simulink model "SG__MDL_IO344"  (R2020a)
settings: Solver=FixedStepDiscrete  StartTime=0.0  StopTime=Inf  RelTol=1e-3  EnableMultiTasking=on
PreLoadFcn:
  | Ts = 0.001;
  | FPGA_Frequency = 75000000;
InitFcn:
  | Ts = 0.001;
  | FPGA_Frequency = 75000000;
libraries: dspfdesign x4, slrtlib x2, SG_library x1, simulink x1, dspsrcs4 x1
settings Model: SimulationMode=external  Creator=lab  LastModifiedBy=padlewsk
settings SolverCC: ConcurrentTasks=on  AutoInsertRateTranBlk=on  InsertRTBMode=Never (minimum delay)
settings DataIOCC: LimitDataPoints=on  SaveFormat=StructureWithTime  SaveOutput=off  SignalLogging=off  DSMLogging=off  SaveTime=off  ReturnWorkspaceOutputs=off
settings OptimizationCC: BlockReduction=off  OptimizeBlockIOStorage=off  BufferReuse=off  GlobalBufferReuse=off  ExpressionFolding=off  LocalBlockOutputs=off  OptimizeDataStoreBuffers=off  BusAssignmentInplaceUpdate=off
settings DebuggingCC: UnconnectedInputMsg=none  UnconnectedOutputMsg=none  UnconnectedLineMsg=none
settings HardwareCC: ProdBitPerPointer=32  ProdBitPerSizeT=32  ProdBitPerPtrDiffT=32  ProdLargestAtomicFloat=None  ProdWordSize=32  ProdLongLongMode=on  ProdHWDeviceType=Generic->32-bit x86 compatible
settings SFSimCC: CustomCodeUndefinedFunction=UseInterfaceOnly
settings RTWCC: Description=Simulink Real-Time  SystemTargetFile=slrt.tlc  TemplateMakefile=slrt_default_tmf  RTWVerbose=off  CodeExecutionProfiling=on  RTWCompilerOptimization=on
settings SimulinkRealTimeCC: SupportVariableSizeSignals=on  xPCConcurrentTasks=on

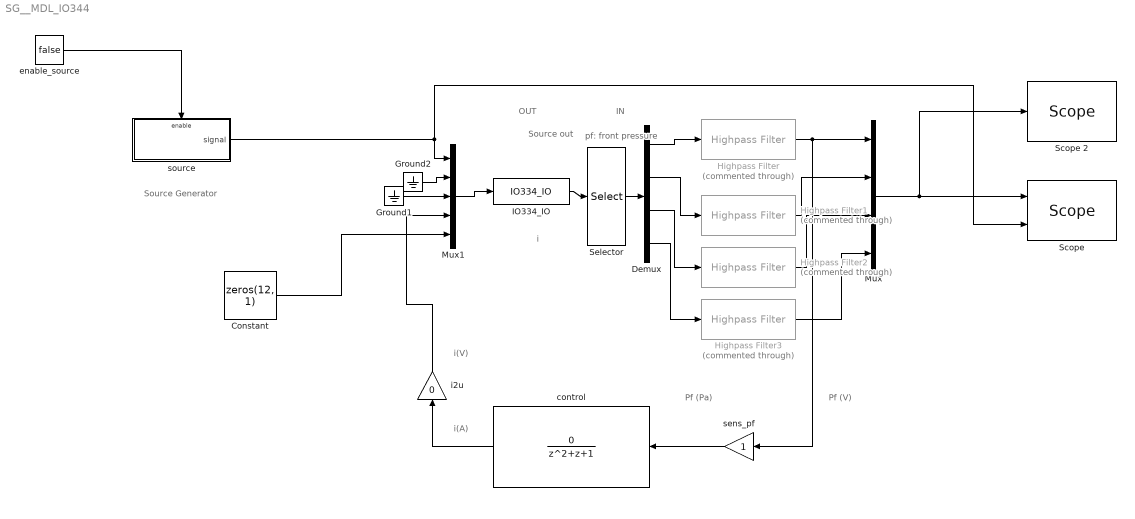
== system SG__MDL_IO344 ==
  note: pf: front pressure
  note: OUT
  note: Source Generator
  note: Source out
  note: IN
  note: i
  note: Pf (V)
  note: i(A)
  note: Pf (Pa)
  note: i(V)
  Constant : Constant  Value=zeros(12, 1)  SampleTime=-1
  Demux : Demux
  Ground1 : Ground
  Ground2 : Ground
  Highpass Filter : dspfdesign/Highpass Filter  Commented=through  FilterType=IIR  DesignForMinimumOrder=off  FilterOrder=4  StopbandFrequency=8e3  PassbandFrequency=5  StopbandAttenuation=80  PassbandRipple=0.1  InheritSampleRate=on  SampleRate=40000  SimulateUsing=Interpreted execution  roundingMode=Floor  coeffsDataTypeStr=fixdt(1,16)
  Highpass Filter1 : dspfdesign/Highpass Filter  Commented=through  FilterType=IIR  DesignForMinimumOrder=off  FilterOrder=4  StopbandFrequency=8e3  PassbandFrequency=5  StopbandAttenuation=80  PassbandRipple=0.1  InheritSampleRate=off  SampleRate=40000  SimulateUsing=Interpreted execution  roundingMode=Floor  coeffsDataTypeStr=fixdt(1,16)
  Highpass Filter2 : dspfdesign/Highpass Filter  Commented=through  FilterType=IIR  DesignForMinimumOrder=off  FilterOrder=4  StopbandFrequency=8e3  PassbandFrequency=5  StopbandAttenuation=80  PassbandRipple=0.1  InheritSampleRate=off  SampleRate=40000  SimulateUsing=Interpreted execution  roundingMode=Floor  coeffsDataTypeStr=fixdt(1,16)
  Highpass Filter3 : dspfdesign/Highpass Filter  Commented=through  FilterType=IIR  DesignForMinimumOrder=on  FilterOrder=50  StopbandFrequency=4  PassbandFrequency=5  StopbandAttenuation=80  PassbandRipple=0.1  InheritSampleRate=off  SampleRate=40000  SimulateUsing=Interpreted execution  roundingMode=Floor  coeffsDataTypeStr=fixdt(1,16)
  IO334_IO : SG_library/Built elements/IO334_IO  ts=ts  OutputRange=± 5V
      settings: SourceProductName=Custom Speedgoat implementations
  Mux : Mux
  Mux1 : Mux  Inputs=5
  "Scope " : slrtlib/Displays and Logging/Scope   scopeno=2  scopetype=Host  autostart=on  viewmode=Graphical redraw  formatstr='%15.6f'  grid=on  ylimits=[0,0]  nosamples=800000  noprepostsamples=0  interleave=1  triggermode=Signal triggering  triggersignal=1  trigsignalfromport=on  triggerlevel=0.0001  triggerslope=Either  triggerscope=1  triggersample=0  filename=data.dat  mode=Lazy  writesize=512  autorestart=off  dynamicfilemode=off  maxwritefilesize=512*1024^2
  Scope 2 : slrtlib/Displays and Logging/Scope   scopeno=1  scopetype=Target  autostart=on  viewmode=Graphical redraw  formatstr='%15.6f'  grid=on  ylimits=[-10,10]  nosamples=800000  noprepostsamples=0  interleave=1  triggermode=FreeRun  triggersignal=1  trigsignalfromport=off  triggerlevel=0.45  triggerslope=Either  triggerscope=1  triggersample=0  filename=data.dat  mode=Lazy  writesize=512  autorestart=off  dynamicfilemode=off  maxwritefilesize=512*1024^2
  Selector : Selector  InputPortWidth=16  IndexOptions=Index vector (dialog)  Indices=1:4  OutputSizes=1
  control : DiscreteTransferFcn  Numerator="[0  0  0]"  Denominator="[1  1  1]"
  enable_source : Constant  Value=false  SampleTime=-1
  i2u : Gain  Gain=0
  sens_pf : Gain
  source : Subsystem  TreatAsAtomicUnit=on
  wires:
  Highpass Filter/1 -> Mux/1, sens_pf/1
  Highpass Filter1/1 -> Mux/2
  Highpass Filter2/1 -> Mux/3
  Highpass Filter3/1 -> Mux/4
  Ground1/1 -> Mux1/3
  Mux/1 -> Scope 2/1, "Scope "/1
  enable_source/1 -> source/Enable
  source/1(signal) -> Mux1/1, "Scope "/2
  Ground2/1 -> Mux1/2
  control/1 -> i2u/1
  sens_pf/1 -> control/1
  i2u/1 -> Mux1/4
  Demux/1 -> Highpass Filter/1
  Demux/2 -> Highpass Filter1/1
  Demux/3 -> Highpass Filter2/1
  Demux/4 -> Highpass Filter3/1
  Mux1/1 -> IO334_IO/1
  Constant/1 -> Mux1/5
  IO334_IO/1 -> Selector/1
  Selector/1 -> Demux/1

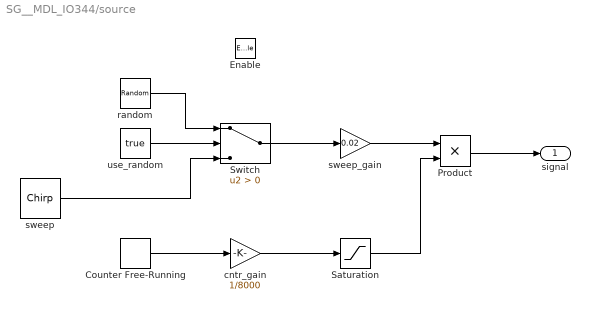
== system SG__MDL_IO344/source ==
  Enable : EnablePort  StatesWhenEnabling=reset
  Counter Free-Running : simulink/Sources/Counter Free-Running  NumBits=32  tsamp=-1
  Product : Product
  Saturation : Saturate  UpperLimit=1  LowerLimit=0
  Switch : Switch  Criteria=u2 > Threshold
  cntr_gain : Gain  Gain=1/8000  ParamDataTypeStr=double
  random : RandomNumber  Variance=0.5  SampleTime=2.5e-05
  sweep : dspsrcs4/Chirp  sweep=Logarithmic  mode=Unidirectional  f0=50  f1=500  t1=5  Tsweep=5  phase=0  Ts=2.5e-05  spf=1  datatype=Double  OutputFrames=off
  sweep_gain : Gain  Gain=0.02
  use_random : Constant  Value=true  SampleTime=-1
  signal : Outport  OutputWhenDisabled=reset  InitialOutput=0  VectorParamsAs1DForOutWhenUnconnected=off
  wires:
  Saturation/1 -> Product/2
  cntr_gain/1 -> Saturation/1
  use_random/1 -> Switch/2
  Counter Free-Running/1 -> cntr_gain/1
  Switch/1 -> sweep_gain/1
  Product/1 -> signal/1
  random/1 -> Switch/1
  sweep_gain/1 -> Product/1
  sweep/1 -> Switch/3
